simulink model "Sender"  (R2014b)
settings: Solver=ode3  StartTime=0.0  StopTime=10  FixedStep=1/5000000  RelTol=1e-3
libraries: commsynccomp2 x1, simulink x1
settings Model: Creator=Eitima  LastModifiedBy=Eitima
settings DataIOCC: ExternalInput=[t,SigTime]  LimitDataPoints=off  LoadExternalInput=on  TimeSaveName=tOut  OutputSaveName=SigTimeOut

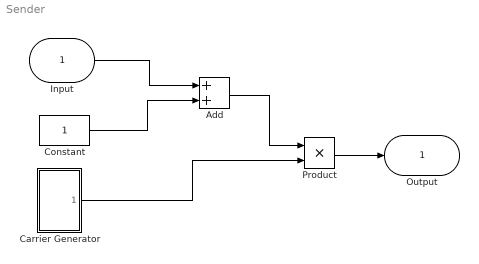
== system Sender ==
  Input : Inport
  Add : Sum
  Carrier Generator : Subsystem
  Constant : Constant
  Product : Product
  Output : Outport
  wires:
  Input/1 -> Add/1
  Constant/1 -> Add/2
  Add/1 -> Product/1
  Carrier Generator/1(Carrier) -> Product/2
  Product/1 -> Output/1

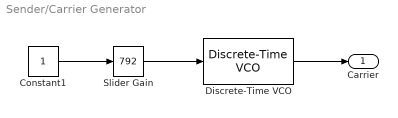
== system Sender/Carrier Generator ==
  Constant1 : Constant
  Discrete-Time VCO : commsynccomp2/Discrete-Time VCO  Ac=1  Fc=0  Kc=1000  Ph=0  ts=1/5000000
  Slider Gain : simulink/Math Operations/Slider Gain  low=550  gain=792  high=1605
  Carrier : Outport
  wires:
  Discrete-Time VCO/1 -> Carrier/1
  Slider Gain/1 -> Discrete-Time VCO/1
  Constant1/1 -> Slider Gain/1
